simulink model "Model_IPS6"  (R2016a)
settings: Solver=VariableStepAuto  StartTime=0  StopTime=15
values from neighbouring files (symbols this model uses):
  Imrn = 7.4    [parametriAM.m]
  In = 12.7    [parametriAM.m]
  Ismax = In*sqrt(2)    [parametriAM.m]
  J = 0.019    [parametriAM.m]
  Ki_Imr = 1000    [parametriAM.m]
  Ki_tok = 5.0    (= 5)    [parametriAM.m]
  Ki_wr = 1000    [parametriAM.m]
  Kp_Imr = 100    [parametriAM.m]
  Kp_tok = 0.05    [parametriAM.m]
  Kp_wr = 50    [parametriAM.m]
  Lm = 0.0493    [parametriAM.m]
  Lr = 0.05315    [parametriAM.m]
  Ls = 0.05315    [parametriAM.m]
  Lst = sigma*Ls    (= 0.00742111947319)    [parametriAM.m]
  pp = 3    [parametriAM.m]
  Rs = 0.594    [parametriAM.m]
  sigma = 1 - 1/((1+sigmaR)*(1+sigmaS))    (= 0.13962595434)    [parametriAM.m]
  taufiltra = 1/(2*pi*fcutoff)    (= 1.59154943092e-05)    [parametriAM.m]
  Tr = Lr/Rr    (= 0.0771407837446)    [parametriAM.m]
  Udc = Un*sqrt(2)    [parametriAM.m]
  wb_upper_limit_field_weaking = sqrt((Ls^2+Lst^2)/(2*Lst^2*Ls^2))*Usmax/Ismax    [parametriAM.m]
  wdod = 2000*2*pi/60    (= 209.439510239)    [parametriAM.m]
libraries: simulink x20
(part 1 of 2)
settings Model: Creator=Vaje  LastModifiedBy=Mitja1

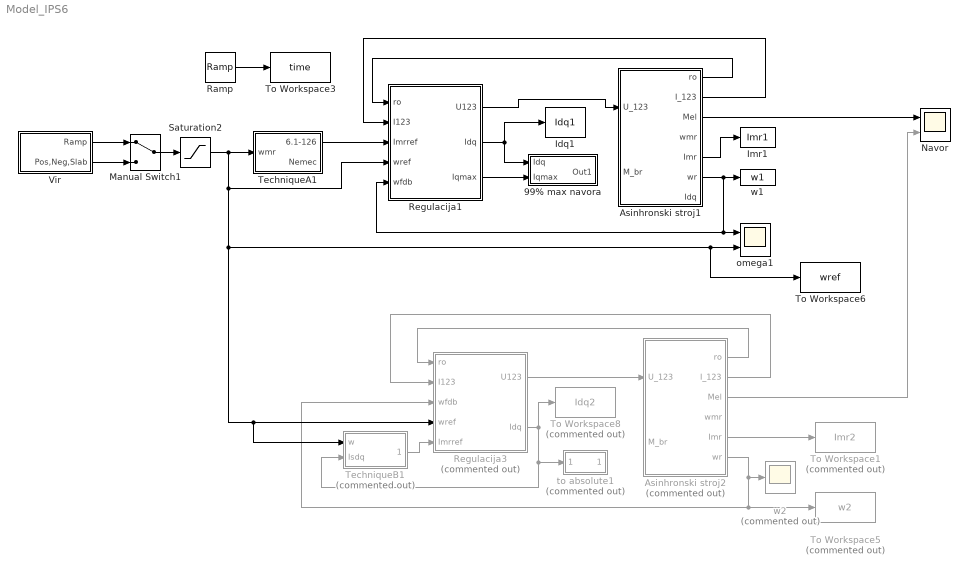
== system Model_IPS6 ==
  99% max navora : Subsystem
  Asinhronski stroj1 : Subsystem  InitFcn=parametriAM
  Asinhronski stroj2 : Subsystem  Commented=on  InitFcn=parametriAM
  Idq1 : ToWorkspace  VariableName=Idq1  SampleTime=-1
      settings: Decimation=3  Save2DSignal=2-D array (concatenate along first dimension)
  Imr1 : ToWorkspace  VariableName=Imr1  SampleTime=-1
      settings: Decimation=3  Save2DSignal=2-D array (concatenate along first dimension)
  Manual Switch1 : ManualSwitch
  Navor : Scope  NumInputPorts=2
  Ramp : simulink/Sources/Ramp  slope=1  start=0  X0=0
  Regulacija1 : Subsystem
  Regulacija3 : Subsystem  Commented=on
  Saturation2 : Saturate  UpperLimit=wb_upper_limit_field_weaking  LowerLimit=-wb_upper_limit_field_weaking
  TechniqueA1 : Subsystem
  TechniqueB1 : Subsystem  Commented=on
  To Workspace1 : ToWorkspace  Commented=on  VariableName=Imr2  SampleTime=-1
      settings: Decimation=3  Save2DSignal=2-D array (concatenate along first dimension)
  To Workspace3 : ToWorkspace  VariableName=time  SampleTime=-1
      settings: Decimation=3  Save2DSignal=2-D array (concatenate along first dimension)
  To Workspace5 : ToWorkspace  Commented=on  VariableName=w2  SampleTime=-1
      settings: Decimation=3  Save2DSignal=2-D array (concatenate along first dimension)
  To Workspace6 : ToWorkspace  VariableName=wref  SampleTime=-1
      settings: Decimation=3  Save2DSignal=2-D array (concatenate along first dimension)
  To Workspace8 : ToWorkspace  Commented=on  VariableName=Idq2  SampleTime=-1
      settings: Decimation=3  Save2DSignal=2-D array (concatenate along first dimension)
  Vir : Subsystem
  omega1 : Scope  NumInputPorts=2
  to absolute1 : Subsystem  Commented=on
  w1 : ToWorkspace  VariableName=w1  SampleTime=-1
      settings: Decimation=3  Save2DSignal=2-D array (concatenate along first dimension)
  w2 : Scope  Commented=on
  wires:
  Vir/1(Ramp) -> Manual Switch1/1
  Vir/2(Pos,Neg,Slab) -> Manual Switch1/2
  Asinhronski stroj1/5(Imr) -> Imr1/1
  Ramp/1 -> To Workspace3/1
  TechniqueA1/1(6.1-126) -> Regulacija1/3(Imrref)
  Regulacija1/2(Idq) -> Idq1/1, 99% max navora/1("\tIdq")
  Asinhronski stroj1/1(ro) -> Regulacija1/1(ro)
  Asinhronski stroj1/2(I_123) -> Regulacija1/2(I123)
  Regulacija1/1(U123) -> Asinhronski stroj1/1(U_123)
  Asinhronski stroj1/6(wr) -> omega1/1, Regulacija1/5(wfdb), w1/1
  Asinhronski stroj2/5(Imr) -> To Workspace1/1
  Manual Switch1/1 -> Saturation2/1
  Regulacija3/2(Idq) -> TechniqueB1/2(Isdq), to absolute1/1(In1), To Workspace8/1
  Asinhronski stroj2/1(ro) -> Regulacija3/1(ro)
  Asinhronski stroj2/2(I_123) -> Regulacija3/2(I123)
  Regulacija3/1(U123) -> Asinhronski stroj2/1(U_123)
  Asinhronski stroj2/6(wr) -> Regulacija3/3(wfdb), To Workspace5/1, w2/1
  TechniqueB1/1(6.1-135) -> Regulacija3/5(Imrref)
  Saturation2/1 -> TechniqueB1/1(w), Regulacija3/4(wref), To Workspace6/1, omega1/2, Regulacija1/4(wref), TechniqueA1/1(wmr)
  Regulacija1/3(Iqmax) -> 99% max navora/2(Iqmax)
  Asinhronski stroj1/3(Mel) -> Navor/1
  Asinhronski stroj2/3(Mel) -> Navor/2

== system Model_IPS6/99% max navora ==
  "\tIdq" : Inport
  Iqmax : Inport  Port=2
  Demux : Demux  Outputs=2
  Gain1 : Gain  Gain=3*pp/2
  Gain2 : Gain  Gain=Lm*Lm/Lr
  Product2 : Product  Inputs=3  RndMeth=Zero
  Step : Step  Time=0.6  After=0.99  SampleTime=0
  Out1 : Outport
  wires:
  "\tIdq"/1 -> Demux/1
  Demux/1 -> Product2/1
  Iqmax/1 -> Product2/2
  Step/1 -> Product2/3
  Gain1/1 -> Gain2/1
  Product2/1 -> Gain1/1
  Gain2/1 -> Out1/1

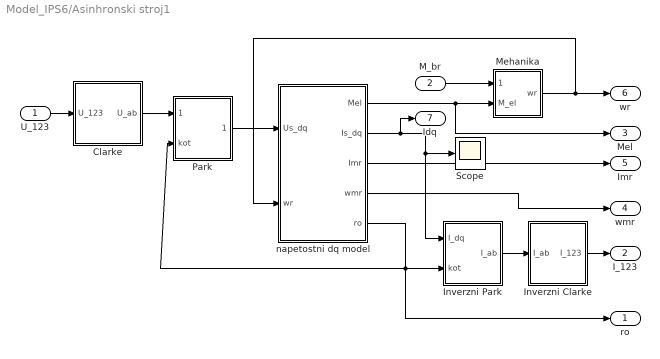
== system Model_IPS6/Asinhronski stroj1 ==
  U_123 : Inport
  M_br : Inport  Port=2
  Clarke : Subsystem
  Inverzni Clarke : Subsystem
  Inverzni Park : Subsystem
  Mehanika : Subsystem
  Park : Subsystem
  Scope : Scope
  napetostni dq model : Subsystem
  ro : Outport
  I_123 : Outport  Port=2
  Mel : Outport  Port=3
  wmr : Outport  Port=4
  Imr : Outport  Port=5
  wr : Outport  Port=6
  Idq : Outport  Port=7
  wires:
  Inverzni Park/1(I_ab) -> Inverzni Clarke/1(I_ab)
  Clarke/1(U_ab) -> Park/1(U_ab)
  Mehanika/1(wr) -> napetostni dq model/2(wr), wr/1
  M_br/1 -> Mehanika/1(M_br)
  napetostni dq model/1(Mel) -> Mel/1, Mehanika/2(M_el)
  Inverzni Clarke/1(I_123) -> I_123/1
  napetostni dq model/4(wmr) -> wmr/1
  napetostni dq model/3(Imr) -> Imr/1
  U_123/1 -> Clarke/1(U_123)
  napetostni dq model/2(Is_dq) -> Idq/1, Scope/1, Inverzni Park/1(I_dq)
  napetostni dq model/5(ro) -> ro/1, Park/2(kot), Inverzni Park/2(kot)
  Park/1(U_dq) -> napetostni dq model/1(Us_dq)

== system Model_IPS6/Asinhronski stroj2 ==
  U_123 : Inport
  M_br : Inport  Port=2
  Clarke : Subsystem
  Inverzni Clarke : Subsystem
  Inverzni Park : Subsystem
  Mehanika : Subsystem
  Park : Subsystem
  Scope : Scope
  napetostni dq model : Subsystem
  ro : Outport
  I_123 : Outport  Port=2
  Mel : Outport  Port=3
  wmr : Outport  Port=4
  Imr : Outport  Port=5
  wr : Outport  Port=6
  wires:
  Park/1(U_dq) -> napetostni dq model/1(Us_dq), Scope/1
  napetostni dq model/5(ro) -> Inverzni Park/2(kot), Park/2(kot), ro/1
  napetostni dq model/2(Is_dq) -> Inverzni Park/1(I_dq)
  U_123/1 -> Clarke/1(U_123)
  napetostni dq model/3(Imr) -> Imr/1
  napetostni dq model/4(wmr) -> wmr/1
  Inverzni Clarke/1(I_123) -> I_123/1
  napetostni dq model/1(Mel) -> Mehanika/2(M_el), Mel/1
  M_br/1 -> Mehanika/1(M_br)
  Mehanika/1(wr) -> wr/1, napetostni dq model/2(wr)
  Clarke/1(U_ab) -> Park/1(U_ab)
  Inverzni Park/1(I_ab) -> Inverzni Clarke/1(I_ab)

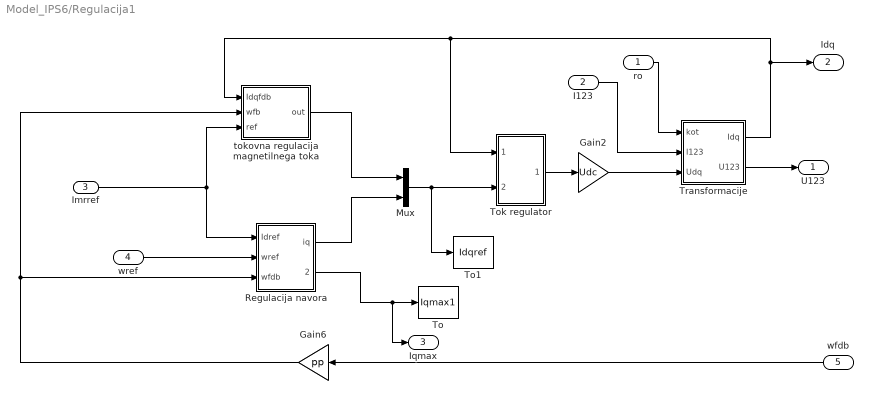
== system Model_IPS6/Regulacija1 ==
  ro : Inport
  I123 : Inport  Port=2
  Imrref : Inport  Port=3
  wref : Inport  Port=4
  wfdb : Inport  Port=5
  Gain2 : Gain  Gain=Udc
  Gain6 : Gain  Gain=pp
  Mux : Mux  Inputs=2
  Regulacija navora : Subsystem
  To : ToWorkspace  VariableName=Iqmax1  SampleTime=-1
      settings: Decimation=3  Save2DSignal=2-D array (concatenate along first dimension)
  To1 : ToWorkspace  VariableName=Idqref  SampleTime=-1
      settings: Decimation=3  Save2DSignal=2-D array (concatenate along first dimension)
  Tok regulator : Subsystem
  Transformacije : Subsystem
  tokovna regulacija magnetilnega toka : Subsystem
  U123 : Outport
  Idq : Outport  Port=2
  Iqmax : Outport  Port=3
  wires:
  Imrref/1 -> Regulacija navora/1(Idref), tokovna regulacija magnetilnega toka/3(ref)
  wref/1 -> Regulacija navora/2(wref)
  Transformacije/1(Idq) -> Tok regulator/1(Idqdej), tokovna regulacija magnetilnega toka/1(Idqfdb), Idq/1
  ro/1 -> Transformacije/1(kot)
  I123/1 -> Transformacije/2(I123)
  Gain2/1 -> Transformacije/3(Udq)
  wfdb/1 -> Gain6/1
  tokovna regulacija magnetilnega toka/1(out) -> Mux/1
  Mux/1 -> To1/1, Tok regulator/2(Idqref)
  Tok regulator/1(Udq) -> Gain2/1
  Regulacija navora/1(iq) -> Mux/2
  Transformacije/2(U123) -> U123/1
  Regulacija navora/2(Iqmax) -> Iqmax/1, To/1
  Gain6/1 -> tokovna regulacija magnetilnega toka/2(wfb), Regulacija navora/3(wfdb)

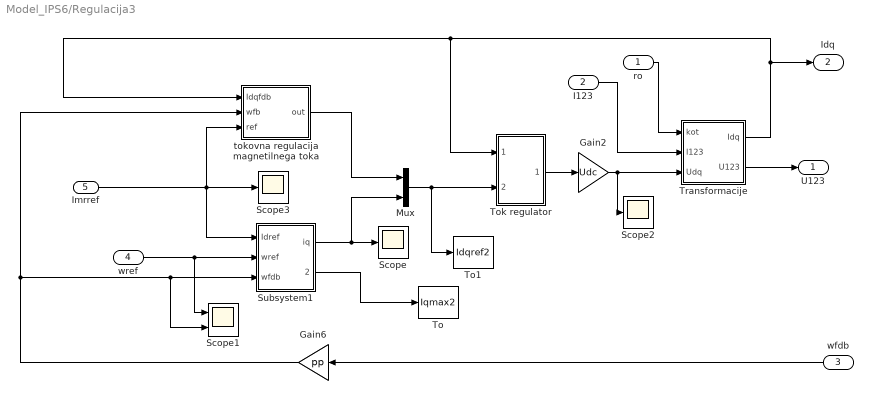
== system Model_IPS6/Regulacija3 ==
  ro : Inport
  I123 : Inport  Port=2
  wfdb : Inport  Port=3
  wref : Inport  Port=4
  Imrref : Inport  Port=5
  Gain2 : Gain  Gain=Udc
  Gain6 : Gain  Gain=pp
  Mux : Mux  Inputs=2
  Scope : Scope
  Scope1 : Scope  NumInputPorts=2
  Scope2 : Scope
  Scope3 : Scope
  Subsystem1 : Subsystem
  To : ToWorkspace  VariableName=Iqmax2  SampleTime=-1
      settings: Decimation=3  Save2DSignal=2-D array (concatenate along first dimension)
  To1 : ToWorkspace  VariableName=Idqref2  SampleTime=-1
      settings: Decimation=3  Save2DSignal=2-D array (concatenate along first dimension)
  Tok regulator : Subsystem
  Transformacije : Subsystem
  tokovna regulacija magnetilnega toka : Subsystem
  U123 : Outport
  Idq : Outport  Port=2
  wires:
  Gain6/1 -> Subsystem1/3(wfdb), Scope1/2, tokovna regulacija magnetilnega toka/2(wfb)
  Subsystem1/2(Iqmax) -> To/1
  Transformacije/2(U123) -> U123/1
  Subsystem1/1(iq) -> Mux/2, Scope/1
  Tok regulator/1(Udq) -> Gain2/1
  Mux/1 -> Tok regulator/2(Idqref), To1/1
  tokovna regulacija magnetilnega toka/1(out) -> Mux/1
  wfdb/1 -> Gain6/1
  Gain2/1 -> Transformacije/3(Udq), Scope2/1
  I123/1 -> Transformacije/2(I123)
  ro/1 -> Transformacije/1(kot)
  Transformacije/1(Idq) -> Idq/1, tokovna regulacija magnetilnega toka/1(Idqfdb), Tok regulator/1(Idqdej)
  wref/1 -> Scope1/1, Subsystem1/2(wref)
  Imrref/1 -> tokovna regulacija magnetilnega toka/3(ref), Scope3/1, Subsystem1/1(Idref)

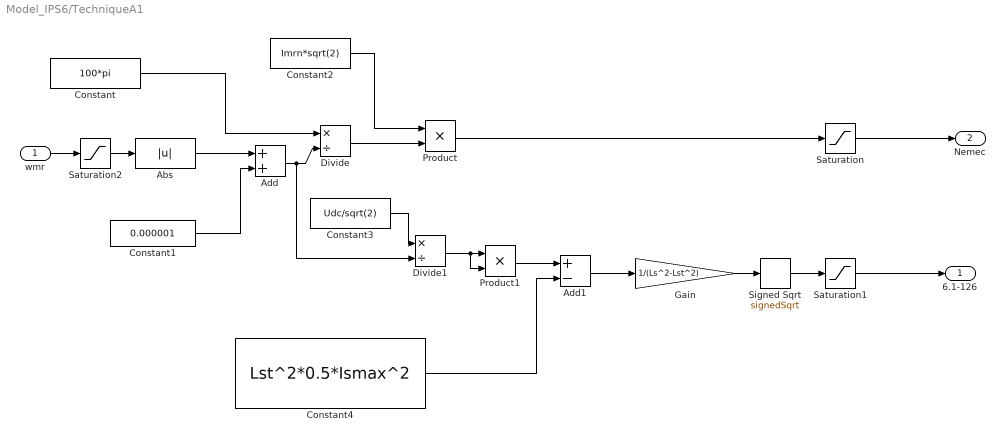
== system Model_IPS6/TechniqueA1 ==
  wmr : Inport
  Abs : Abs
  Add : Sum
  Add1 : Sum  Inputs=+-
  Constant : Constant  Value=100*pi
  Constant1 : Constant  Value=0.000001
  Constant2 : Constant  Value=Imrn*sqrt(2)
  Constant3 : Constant  Value=Udc/sqrt(2)
  Constant4 : Constant  Value=Lst^2*0.5*Ismax^2
  Divide : Product  Inputs=*/
  Divide1 : Product  Inputs=*/
  Gain : Gain  Gain=1/(Ls^2-Lst^2)
  Product : Product
  Product1 : Product
  Saturation : Saturate  UpperLimit=+Imrn*sqrt(2)  LowerLimit=0
  Saturation1 : Saturate  UpperLimit=+Imrn*sqrt(2)  LowerLimit=-Imrn*sqrt(2)
  Saturation2 : Saturate  UpperLimit=wb_upper_limit_field_weaking  LowerLimit=-wb_upper_limit_field_weaking
  Signed Sqrt : Sqrt  Operator=signedSqrt  SaturateOnIntegerOverflow=on
  6.1-126 : Outport
  Nemec : Outport  Port=2
  wires:
  Constant2/1 -> Product/1
  Divide/1 -> Product/2
  Product/1 -> Saturation/1
  Constant/1 -> Divide/1
  Add/1 -> Divide1/2, Divide/2
  Abs/1 -> Add/1
  Constant1/1 -> Add/2
  Saturation/1 -> Nemec/1
  Constant3/1 -> Divide1/1
  Divide1/1 -> Product1/2, Product1/1
  Product1/1 -> Add1/1
  Constant4/1 -> Add1/2
  Saturation1/1 -> 6.1-126/1
  Add1/1 -> Gain/1
  Gain/1 -> Signed Sqrt/1
  Signed Sqrt/1 -> Saturation1/1
  wmr/1 -> Saturation2/1
  Saturation2/1 -> Abs/1

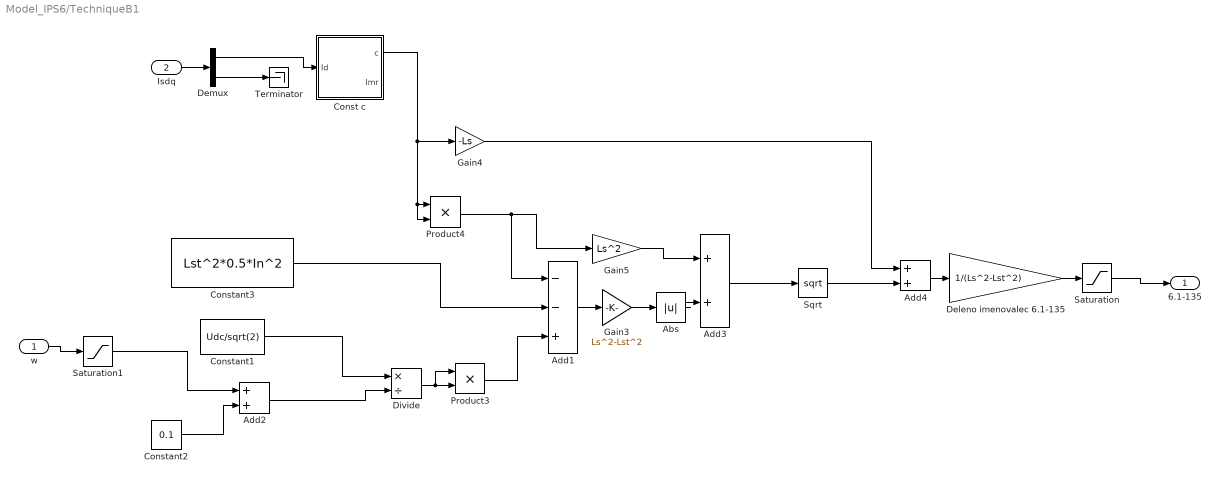
== system Model_IPS6/TechniqueB1 ==
  w : Inport
  Isdq : Inport  Port=2
  Abs : Abs
  Add1 : Sum  Inputs=--+
  Add2 : Sum
  Add3 : Sum
  Add4 : Sum
  Const c : Subsystem
  Constant1 : Constant  Value=Udc/sqrt(2)
  Constant2 : Constant  Value=0.1
  Constant3 : Constant  Value=Lst^2*0.5*In^2
  Deleno imenovalec 6.1-135 : Gain  Gain=1/(Ls^2-Lst^2)
  Demux : Demux  Outputs=2
  Divide : Product  Inputs=*/
  Gain3 : Gain  Gain=Ls^2-Lst^2
  Gain4 : Gain  Gain=-Ls
  Gain5 : Gain  Gain=Ls^2
  Product3 : Product
  Product4 : Product
  Saturation : Saturate  UpperLimit=+Imrn*sqrt(2)  LowerLimit=-Imrn*sqrt(2)
  Saturation1 : Saturate  UpperLimit=wb_upper_limit_field_weaking  LowerLimit=-wb_upper_limit_field_weaking
  Sqrt : Sqrt  SaturateOnIntegerOverflow=on
  Terminator : Terminator
  6.1-135 : Outport
  wires:
  Constant1/1 -> Divide/1
  w/1 -> Saturation1/1
  Constant2/1 -> Add2/2
  Demux/1 -> Const c/1(Id)
  Demux/2 -> Terminator/1
  Saturation/1 -> 6.1-135/1
  Const c/1(c) -> Product4/2, Product4/1, Gain4/1
  Product4/1 -> Add1/1, Gain5/1
  Gain5/1 -> Add3/1
  Gain4/1 -> Add4/1
  Add4/1 -> Deleno imenovalec 6.1-135/1
  Deleno imenovalec 6.1-135/1 -> Saturation/1
  Add1/1 -> Gain3/1
  Constant3/1 -> Add1/2
  Add2/1 -> Divide/2
  Divide/1 -> Product3/1, Product3/2
  Product3/1 -> Add1/3
  Sqrt/1 -> Add4/2
  Gain3/1 -> Abs/1
  Add3/1 -> Sqrt/1
  Abs/1 -> Add3/2
  Saturation1/1 -> Add2/1
  Isdq/1 -> Demux/1

== system Model_IPS6/Vir ==
  Add1 : Sum  Inputs=++++++
  Rampa : simulink/Sources/Ramp  slope=500*2*pi/60  start=0.5  X0=0
  Step : Step  Time=0.2  After=2000*2*pi/60  SampleTime=0
  Step1 : Step  Time=0.4  After=1000*pi/30  SampleTime=0
  Step2 : Step  Time=2  After=2000*2*pi/60  SampleTime=0
  Step3 : Step  Time=3  After=2000*2*pi/60  SampleTime=0
  Step4 : Step  Time=8  After=wdod  SampleTime=0
  Step5 : Step  Time=9  After=wdod  SampleTime=0
  Ramp : Outport
  Pos,Neg,Slab : Outport  Port=2
  wires:
  Add1/1 -> Pos,Neg,Slab/1
  Step/1 -> Add1/1
  Rampa/1 -> Ramp/1
  Step1/1 -> Add1/2

== system Model_IPS6/to absolute1 ==
  In1 : Inport
  Abs1 : Abs
  Demux : Demux  Outputs=2
  Real-Imag to Complex1 : RealImagToComplex
  Out1 : Outport
  wires:
  Demux/2 -> Real-Imag to Complex1/2
  Demux/1 -> Real-Imag to Complex1/1
  In1/1 -> Demux/1
  Abs1/1 -> Out1/1
  Real-Imag to Complex1/1 -> Abs1/1

== system Model_IPS6/Asinhronski stroj1/Clarke ==
  U_123 : Inport
  ABC_ab1 : Subsystem
  Demux : Demux  Outputs=3
  Mux : Mux  Inputs=2
  U_ab : Outport
  wires:
  Mux/1 -> U_ab/1
  ABC_ab1/2(beta) -> Mux/2
  ABC_ab1/1(alfa) -> Mux/1
  Demux/3 -> ABC_ab1/3(C)
  Demux/2 -> ABC_ab1/2(B)
  Demux/1 -> ABC_ab1/1(A)
  U_123/1 -> Demux/1

== system Model_IPS6/Asinhronski stroj1/Inverzni Clarke ==
  I_ab : Inport
  Demux : Demux  Outputs=2
  Mux : Mux  Inputs=3
  ab_ABC : Subsystem
  I_123 : Outport
  wires:
  ab_ABC/3(C) -> Mux/3
  ab_ABC/2(B) -> Mux/2
  ab_ABC/1(A) -> Mux/1
  Demux/2 -> ab_ABC/2(beta)
  Demux/1 -> ab_ABC/1(alfa)
  I_ab/1 -> Demux/1
  Mux/1 -> I_123/1

== system Model_IPS6/Asinhronski stroj1/Inverzni Park ==
  I_dq : Inport
  kot : Inport  Port=2
  Demux : Demux  Outputs=2
  Mux : Mux  Inputs=2
  "Sum1 " : Sum  Inputs=+-  SaturateOnIntegerOverflow=on  InputSameDT=on  OutDataTypeStr=Inherit: Same as first input
  Sum2 : Sum  SaturateOnIntegerOverflow=on  InputSameDT=on  OutDataTypeStr=Inherit: Same as first input
  cos : Fcn  Expr=cos(u)
  sin : Fcn  Expr=sin(u)
  x_d*cos : Product  SaturateOnIntegerOverflow=on  RndMeth=Zero  InputSameDT=on  OutDataTypeStr=Inherit: Same as first input
  x_d*sin : Product  SaturateOnIntegerOverflow=on  RndMeth=Zero  InputSameDT=on  OutDataTypeStr=Inherit: Same as first input
  x_q*cos : Product  SaturateOnIntegerOverflow=on  RndMeth=Zero  InputSameDT=on  OutDataTypeStr=Inherit: Same as first input
  "x_q*sin " : Product  SaturateOnIntegerOverflow=on  RndMeth=Zero  InputSameDT=on  OutDataTypeStr=Inherit: Same as first input
  I_ab : Outport
  wires:
  Mux/1 -> I_ab/1
  I_dq/1 -> Demux/1
  Demux/1 -> x_d*sin/1, x_d*cos/1
  Demux/2 -> "x_q*sin "/1, x_q*cos/1
  cos/1 -> x_q*cos/2, x_d*cos/2
  sin/1 -> "x_q*sin "/2, x_d*sin/2
  x_d*cos/1 -> "Sum1 "/1
  "x_q*sin "/1 -> "Sum1 "/2
  x_q*cos/1 -> Sum2/2
  x_d*sin/1 -> Sum2/1
  "Sum1 "/1 -> Mux/1
  Sum2/1 -> Mux/2
  kot/1 -> cos/1, sin/1

== system Model_IPS6/Asinhronski stroj1/Mehanika ==
  M_br : Inport
  M_el : Inport  Port=2
  Sum : Sum  Inputs=+-
  eq 2.19 : Subsystem
  wr : Outport
  wires:
  M_br/1 -> Sum/2
  Sum/1 -> eq 2.19/1(M)
  M_el/1 -> Sum/1
  eq 2.19/1(wr) -> wr/1

== system Model_IPS6/Asinhronski stroj1/Park ==
  U_ab : Inport
  kot : Inport  Port=2
  Demux : Demux  Outputs=2
  Mux : Mux  Inputs=2
  "Sum1 " : Sum  SaturateOnIntegerOverflow=on  InputSameDT=on  OutDataTypeStr=Inherit: Same as first input
  Sum2 : Sum  Inputs=-+  SaturateOnIntegerOverflow=on  InputSameDT=on  OutDataTypeStr=Inherit: Same as first input
  cos : Fcn  Expr=cos(u)
  sin : Fcn  Expr=sin(u)
  x_a*cos : Product  SaturateOnIntegerOverflow=on  RndMeth=Zero  InputSameDT=on  OutDataTypeStr=Inherit: Same as first input
  x_a*sin : Product  SaturateOnIntegerOverflow=on  RndMeth=Zero  InputSameDT=on  OutDataTypeStr=Inherit: Same as first input
  x_b*cos : Product  SaturateOnIntegerOverflow=on  RndMeth=Zero  InputSameDT=on  OutDataTypeStr=Inherit: Same as first input
  "x_b*sin " : Product  SaturateOnIntegerOverflow=on  RndMeth=Zero  InputSameDT=on  OutDataTypeStr=Inherit: Same as first input
  U_dq : Outport
  wires:
  Mux/1 -> U_dq/1
  U_ab/1 -> Demux/1
  Demux/1 -> x_a*sin/1, x_a*cos/1
  Demux/2 -> "x_b*sin "/1, x_b*cos/1
  cos/1 -> x_b*cos/2, x_a*cos/2
  sin/1 -> "x_b*sin "/2, x_a*sin/2
  x_a*cos/1 -> "Sum1 "/1
  "x_b*sin "/1 -> "Sum1 "/2
  x_b*cos/1 -> Sum2/2
  x_a*sin/1 -> Sum2/1
  "Sum1 "/1 -> Mux/1
  Sum2/1 -> Mux/2
  kot/1 -> cos/1, sin/1

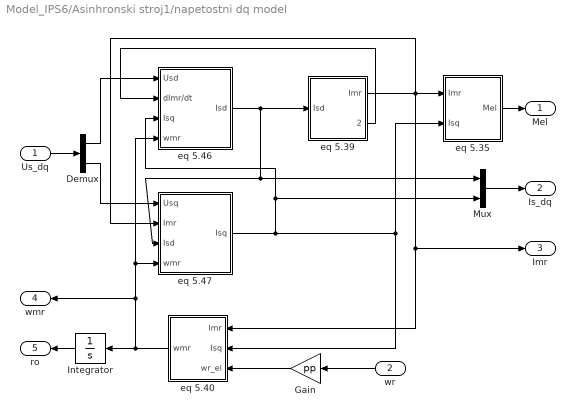
== system Model_IPS6/Asinhronski stroj1/napetostni dq model ==
  Us_dq : Inport
  wr : Inport  Port=2
  Demux : Demux  Outputs=2
  Gain : Gain  Gain=pp
  Integrator : Integrator
  Mux : Mux  Inputs=2
  eq 5.35 : Subsystem
  eq 5.39 : Subsystem
  eq 5.40 : Subsystem
  eq 5.46 : Subsystem
  eq 5.47 : Subsystem
  Mel : Outport
  Is_dq : Outport  Port=2
  Imr : Outport  Port=3
  wmr : Outport  Port=4
  ro : Outport  Port=5
  wires:
  Gain/1 -> eq 5.40/3(wr_el)
  Mux/1 -> Is_dq/1
  Demux/2 -> eq 5.47/1(Usq)
  Demux/1 -> eq 5.46/1(Usd)
  Us_dq/1 -> Demux/1
  wr/1 -> Gain/1
  Integrator/1 -> ro/1
  eq 5.35/1(Mel) -> Mel/1
  eq 5.40/1(wmr) -> Integrator/1, wmr/1, eq 5.46/4(wmr), eq 5.47/4(wmr)
  eq 5.47/1(Isq) -> Mux/2, eq 5.46/3(Isq), eq 5.40/2(Isq), eq 5.35/2(Isq)
  eq 5.39/1(Imr) -> eq 5.47/2(Imr), Imr/1, eq 5.40/1(Imr), eq 5.35/1(Imr)
  eq 5.39/2(dImr/dt) -> eq 5.46/2(dImr/dt)
  eq 5.46/1(Isd) -> Mux/1, eq 5.47/3(Isd), eq 5.39/1(Isd)

== system Model_IPS6/Asinhronski stroj2/Clarke ==
  U_123 : Inport
  ABC_ab1 : Subsystem
  Demux : Demux  Outputs=3
  Mux : Mux  Inputs=2
  U_ab : Outport
  wires:
  U_123/1 -> Demux/1
  Demux/1 -> ABC_ab1/1(A)
  Demux/2 -> ABC_ab1/2(B)
  Demux/3 -> ABC_ab1/3(C)
  ABC_ab1/1(alfa) -> Mux/1
  ABC_ab1/2(beta) -> Mux/2
  Mux/1 -> U_ab/1

== system Model_IPS6/Asinhronski stroj2/Inverzni Clarke ==
  I_ab : Inport
  Demux : Demux  Outputs=2
  Mux : Mux  Inputs=3
  ab_ABC : Subsystem
  I_123 : Outport
  wires:
  Mux/1 -> I_123/1
  I_ab/1 -> Demux/1
  Demux/1 -> ab_ABC/1(alfa)
  Demux/2 -> ab_ABC/2(beta)
  ab_ABC/1(A) -> Mux/1
  ab_ABC/2(B) -> Mux/2
  ab_ABC/3(C) -> Mux/3

== system Model_IPS6/Asinhronski stroj2/Inverzni Park ==
  I_dq : Inport
  kot : Inport  Port=2
  Demux : Demux  Outputs=2
  Mux : Mux  Inputs=2
  "Sum1 " : Sum  Inputs=+-  SaturateOnIntegerOverflow=on  InputSameDT=on  OutDataTypeStr=Inherit: Same as first input
  Sum2 : Sum  SaturateOnIntegerOverflow=on  InputSameDT=on  OutDataTypeStr=Inherit: Same as first input
  cos : Fcn  Expr=cos(u)
  sin : Fcn  Expr=sin(u)
  x_d*cos : Product  SaturateOnIntegerOverflow=on  RndMeth=Zero  InputSameDT=on  OutDataTypeStr=Inherit: Same as first input
  x_d*sin : Product  SaturateOnIntegerOverflow=on  RndMeth=Zero  InputSameDT=on  OutDataTypeStr=Inherit: Same as first input
  x_q*cos : Product  SaturateOnIntegerOverflow=on  RndMeth=Zero  InputSameDT=on  OutDataTypeStr=Inherit: Same as first input
  "x_q*sin " : Product  SaturateOnIntegerOverflow=on  RndMeth=Zero  InputSameDT=on  OutDataTypeStr=Inherit: Same as first input
  I_ab : Outport
  wires:
  kot/1 -> sin/1, cos/1
  Sum2/1 -> Mux/2
  "Sum1 "/1 -> Mux/1
  x_d*sin/1 -> Sum2/1
  x_q*cos/1 -> Sum2/2
  "x_q*sin "/1 -> "Sum1 "/2
  x_d*cos/1 -> "Sum1 "/1
  sin/1 -> x_d*sin/2, "x_q*sin "/2
  cos/1 -> x_d*cos/2, x_q*cos/2
  Demux/2 -> x_q*cos/1, "x_q*sin "/1
  Demux/1 -> x_d*cos/1, x_d*sin/1
  I_dq/1 -> Demux/1
  Mux/1 -> I_ab/1

== system Model_IPS6/Asinhronski stroj2/Mehanika ==
  M_br : Inport
  M_el : Inport  Port=2
  Sum : Sum  Inputs=+-
  eq 2.19 : Subsystem
  wr : Outport
  wires:
  eq 2.19/1(wr) -> wr/1
  M_el/1 -> Sum/1
  Sum/1 -> eq 2.19/1(M)
  M_br/1 -> Sum/2

== system Model_IPS6/Asinhronski stroj2/Park ==
  U_ab : Inport
  kot : Inport  Port=2
  Demux : Demux  Outputs=2
  Mux : Mux  Inputs=2
  "Sum1 " : Sum  SaturateOnIntegerOverflow=on  InputSameDT=on  OutDataTypeStr=Inherit: Same as first input
  Sum2 : Sum  Inputs=-+  SaturateOnIntegerOverflow=on  InputSameDT=on  OutDataTypeStr=Inherit: Same as first input
  cos : Fcn  Expr=cos(u)
  sin : Fcn  Expr=sin(u)
  x_a*cos : Product  SaturateOnIntegerOverflow=on  RndMeth=Zero  InputSameDT=on  OutDataTypeStr=Inherit: Same as first input
  x_a*sin : Product  SaturateOnIntegerOverflow=on  RndMeth=Zero  InputSameDT=on  OutDataTypeStr=Inherit: Same as first input
  x_b*cos : Product  SaturateOnIntegerOverflow=on  RndMeth=Zero  InputSameDT=on  OutDataTypeStr=Inherit: Same as first input
  "x_b*sin " : Product  SaturateOnIntegerOverflow=on  RndMeth=Zero  InputSameDT=on  OutDataTypeStr=Inherit: Same as first input
  U_dq : Outport
  wires:
  kot/1 -> sin/1, cos/1
  Sum2/1 -> Mux/2
  "Sum1 "/1 -> Mux/1
  x_a*sin/1 -> Sum2/1
  x_b*cos/1 -> Sum2/2
  "x_b*sin "/1 -> "Sum1 "/2
  x_a*cos/1 -> "Sum1 "/1
  sin/1 -> x_a*sin/2, "x_b*sin "/2
  cos/1 -> x_a*cos/2, x_b*cos/2
  Demux/2 -> x_b*cos/1, "x_b*sin "/1
  Demux/1 -> x_a*cos/1, x_a*sin/1
  U_ab/1 -> Demux/1
  Mux/1 -> U_dq/1

== system Model_IPS6/Asinhronski stroj2/napetostni dq model ==
  Us_dq : Inport
  wr : Inport  Port=2
  Demux : Demux  Outputs=2
  Gain : Gain  Gain=pp
  Integrator : Integrator
  Mux : Mux  Inputs=2
  eq 5.35 : Subsystem
  eq 5.39 : Subsystem
  eq 5.40 : Subsystem
  eq 5.46 : Subsystem
  eq 5.47 : Subsystem
  Mel : Outport
  Is_dq : Outport  Port=2
  Imr : Outport  Port=3
  wmr : Outport  Port=4
  ro : Outport  Port=5
  wires:
  eq 5.46/1(Isd) -> eq 5.39/1(Isd), eq 5.47/3(Isd), Mux/1
  eq 5.39/2(dImr/dt) -> eq 5.46/2(dImr/dt)
  eq 5.39/1(Imr) -> eq 5.35/1(Imr), eq 5.40/1(Imr), Imr/1, eq 5.47/2(Imr)
  eq 5.47/1(Isq) -> eq 5.35/2(Isq), eq 5.40/2(Isq), eq 5.46/3(Isq), Mux/2
  eq 5.40/1(wmr) -> eq 5.47/4(wmr), eq 5.46/4(wmr), wmr/1, Integrator/1
  eq 5.35/1(Mel) -> Mel/1
  Integrator/1 -> ro/1
  wr/1 -> Gain/1
  Us_dq/1 -> Demux/1
  Demux/1 -> eq 5.46/1(Usd)
  Demux/2 -> eq 5.47/1(Usq)
  Mux/1 -> Is_dq/1
  Gain/1 -> eq 5.40/3(wr_el)

== system Model_IPS6/Regulacija1/Regulacija navora ==
  Idref : Inport
  wref : Inport  Port=2
  wfdb : Inport  Port=3
  1/Ti : Gain  Gain=Ki_wr  SaturateOnIntegerOverflow=on  OutDataTypeStr=Inherit: Same as input  ParamDataTypeStr=Inherit: Same as input
  Abs : Abs
  Add2 : Sum  Inputs=+-
  Compare To Zero : simulink/Logic and Bit Operations/Compare To Zero  relop=<=  OutDataTypeStr=boolean
  Integrator : Integrator
  Kp : Gain  Gain=Kp_wr  SaturateOnIntegerOverflow=on  OutDataTypeStr=Inherit: Same as input  ParamDataTypeStr=Inherit: Same as input
  Limita q toka : Subsystem
  Product : Product
  Sum1 : Sum  Inputs=|+-
  Sum2 : Sum  Inputs=|++
  iq : Outport
  Iqmax : Outport  Port=2
  wires:
  1/Ti/1 -> Integrator/1
  Sum1/1 -> Product/1, Kp/1
  Integrator/1 -> Sum2/2
  Add2/1 -> Abs/1
  Abs/1 -> Compare To Zero/1
  Kp/1 -> Sum2/1
  Compare To Zero/1 -> Product/2
  Product/1 -> 1/Ti/1
  wref/1 -> Sum1/1
  wfdb/1 -> Limita q toka/2(w), Sum1/2
  Sum2/1 -> Limita q toka/3(Iq), Add2/1
  Limita q toka/2(Iq_lim) -> Add2/2, iq/1
  Idref/1 -> Limita q toka/1(Idref)
  Limita q toka/1(Out1) -> Iqmax/1

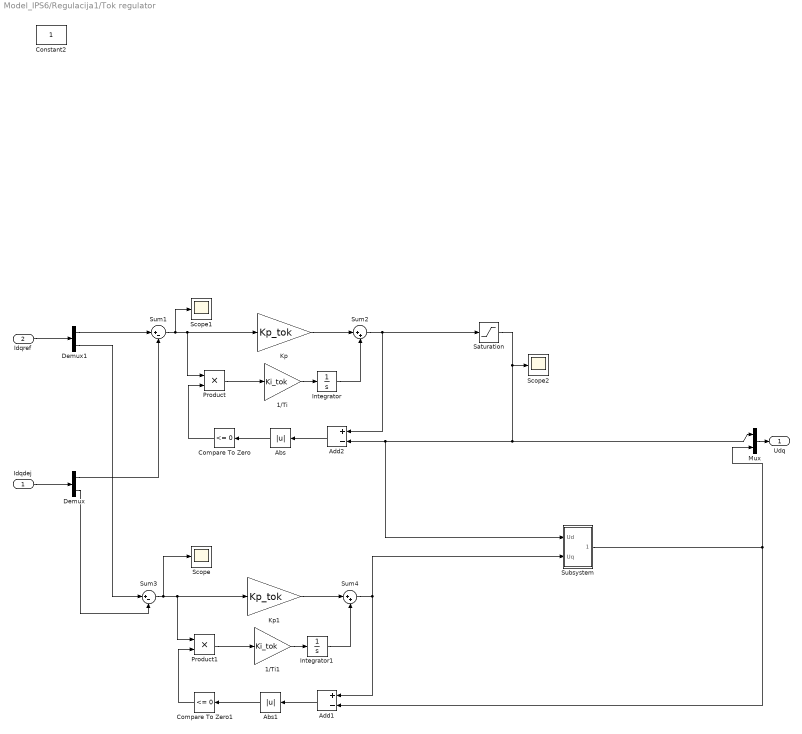
== system Model_IPS6/Regulacija1/Tok regulator ==
  Idqdej : Inport
  Idqref : Inport  Port=2
  1/Ti : Gain  Gain=Ki_tok  SaturateOnIntegerOverflow=on  OutDataTypeStr=Inherit: Same as input  ParamDataTypeStr=Inherit: Same as input
  1/Ti1 : Gain  Gain=Ki_tok  SaturateOnIntegerOverflow=on  OutDataTypeStr=Inherit: Same as input  ParamDataTypeStr=Inherit: Same as input
  Abs : Abs  ZeroCross=off
  Abs1 : Abs
  Add1 : Sum  Inputs=+-
  Add2 : Sum  Inputs=+-
  Compare To Zero : simulink/Logic and Bit Operations/Compare To Zero  relop=<=  OutDataTypeStr=boolean  ZeroCross=off
  Compare To Zero1 : simulink/Logic and Bit Operations/Compare To Zero  relop=<=  OutDataTypeStr=boolean
  Constant2 : Constant
  Demux : Demux  Outputs=2
  Demux1 : Demux  Outputs=2
  Integrator : Integrator
  Integrator1 : Integrator
  Kp : Gain  Gain=Kp_tok  SaturateOnIntegerOverflow=on  OutDataTypeStr=Inherit: Same as input  ParamDataTypeStr=Inherit: Same as input
  Kp1 : Gain  Gain=Kp_tok  SaturateOnIntegerOverflow=on  OutDataTypeStr=Inherit: Same as input  ParamDataTypeStr=Inherit: Same as input
  Mux : Mux  Inputs=2
  Product : Product
  Product1 : Product
  Saturation : Saturate  UpperLimit=0.990  LowerLimit=-0.990  ZeroCross=off
  Scope : Scope
  Scope1 : Scope
  Scope2 : Scope
  Subsystem : Subsystem
  Sum1 : Sum  Inputs=|+-
  Sum2 : Sum  Inputs=|++
  Sum3 : Sum  Inputs=|+-
  Sum4 : Sum  Inputs=|++
  Udq : Outport
  wires:
  Abs1/1 -> Compare To Zero1/1
  Add1/1 -> Abs1/1
  Compare To Zero1/1 -> Product1/2
  Product1/1 -> 1/Ti1/1
  Integrator1/1 -> Sum4/2
  Kp1/1 -> Sum4/1
  1/Ti1/1 -> Integrator1/1
  Sum3/1 -> Scope/1, Kp1/1, Product1/1
  Demux1/2 -> Sum3/1
  Idqref/1 -> Demux1/1
  Mux/1 -> Udq/1
  Sum1/1 -> Scope1/1, Product/1, Kp/1
  Integrator/1 -> Sum2/2
  Kp/1 -> Sum2/1
  Demux1/1 -> Sum1/1
  1/Ti/1 -> Integrator/1
  Add2/1 -> Abs/1
  Abs/1 -> Compare To Zero/1
  Compare To Zero/1 -> Product/2
  Product/1 -> 1/Ti/1
  Idqdej/1 -> Demux/1
  Demux/2 -> Sum3/2
  Demux/1 -> Sum1/2
  Saturation/1 -> Scope2/1, Mux/1, Subsystem/1(Ud), Add2/2
  Sum4/1 -> Add1/1, Subsystem/2(Uq)
  Sum2/1 -> Saturation/1, Add2/1
  Subsystem/1(Uq_lim) -> Add1/2, Mux/2

== system Model_IPS6/Regulacija1/Transformacije ==
  kot : Inport
  I123 : Inport  Port=2
  Udq : Inport  Port=3
  Clarke : Subsystem
  Inverzni Clarke : Subsystem
  Inverzni Park : Subsystem
  Park : Subsystem
  Idq : Outport
  U123 : Outport  Port=2
  wires:
  Inverzni Clarke/1(U_123) -> U123/1
  Park/1(I_dq) -> Idq/1
  kot/1 -> Park/2(kot), Inverzni Park/1(kot)
  Clarke/1(I_ab) -> Park/1(I_ab)
  Inverzni Park/1(U_ab) -> Inverzni Clarke/1(U_ab)
  Udq/1 -> Inverzni Park/2(U_dq)
  I123/1 -> Clarke/1(I_123)

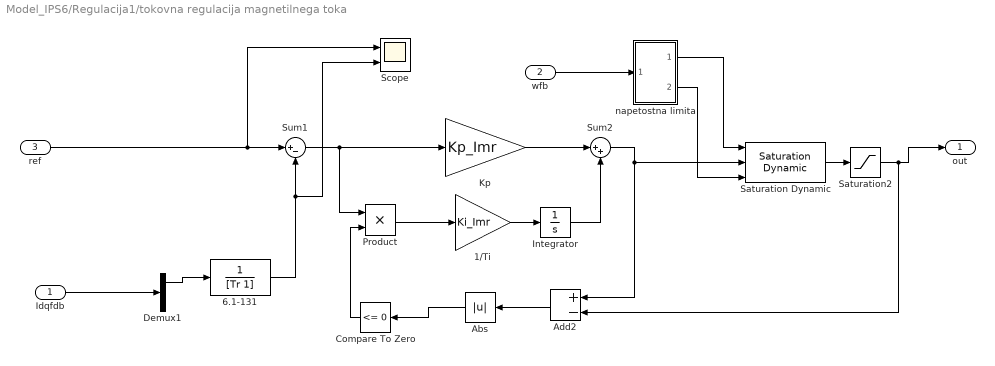
== system Model_IPS6/Regulacija1/tokovna regulacija magnetilnega toka ==
  Idqfdb : Inport
  wfb : Inport  Port=2
  ref : Inport  Port=3
  1/Ti : Gain  Gain=Ki_Imr  SaturateOnIntegerOverflow=on  OutDataTypeStr=Inherit: Same as input  ParamDataTypeStr=Inherit: Same as input
  6.1-131 : TransferFcn  Denominator=[Tr 1]
  Abs : Abs
  Add2 : Sum  Inputs=+-
  Compare To Zero : simulink/Logic and Bit Operations/Compare To Zero  relop=<=  OutDataTypeStr=boolean
  Demux1 : Demux  Outputs=2
  Integrator : Integrator
  Kp : Gain  Gain=Kp_Imr  SaturateOnIntegerOverflow=on  OutDataTypeStr=Inherit: Same as input  ParamDataTypeStr=Inherit: Same as input
  Product : Product
  Saturation Dynamic : simulink/Discontinuities/Saturation Dynamic  OutMin=[]  OutMax=[]  OutDataTypeStr=Inherit: Same as second input  OutDataType=fixdt(1, 16)  OutScaling=2^-10  DoSatur=off
  Saturation2 : Saturate  UpperLimit=Ismax  LowerLimit=-Ismax
  Scope : Scope  NumInputPorts=2
  Sum1 : Sum  Inputs=|+-
  Sum2 : Sum  Inputs=|++
  napetostna limita : Subsystem
  out : Outport
  wires:
  Product/1 -> 1/Ti/1
  Compare To Zero/1 -> Product/2
  Abs/1 -> Compare To Zero/1
  Add2/1 -> Abs/1
  Sum2/1 -> Add2/1, Saturation Dynamic/2
  Integrator/1 -> Sum2/2
  ref/1 -> Scope/1, Sum1/1
  Sum1/1 -> Kp/1, Product/1
  1/Ti/1 -> Integrator/1
  Kp/1 -> Sum2/1
  Demux1/1 -> 6.1-131/1
  6.1-131/1 -> Scope/2, Sum1/2
  Idqfdb/1 -> Demux1/1
  wfb/1 -> napetostna limita/1(wfb)
  napetostna limita/1(Out1) -> Saturation Dynamic/1
  napetostna limita/2(Out2) -> Saturation Dynamic/3
  Saturation Dynamic/1 -> Saturation2/1
  Saturation2/1 -> Add2/2, out/1

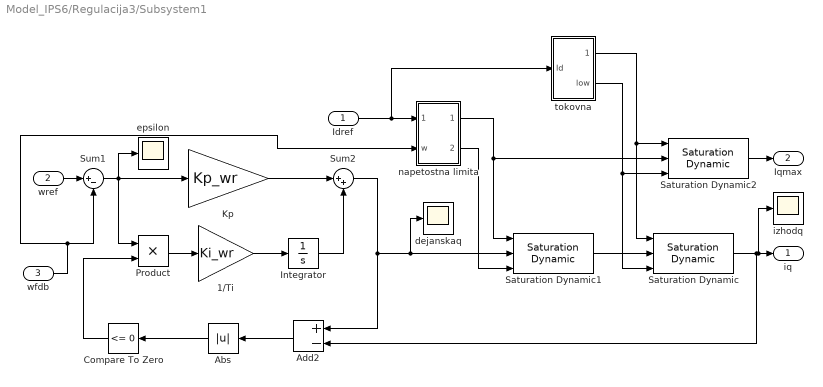
== system Model_IPS6/Regulacija3/Subsystem1 ==
  Idref : Inport
  wref : Inport  Port=2
  wfdb : Inport  Port=3
  1/Ti : Gain  Gain=Ki_wr  SaturateOnIntegerOverflow=on  OutDataTypeStr=Inherit: Same as input  ParamDataTypeStr=Inherit: Same as input
  Abs : Abs
  Add2 : Sum  Inputs=+-
  Compare To Zero : simulink/Logic and Bit Operations/Compare To Zero  relop=<=  OutDataTypeStr=boolean
  Integrator : Integrator
  Kp : Gain  Gain=Kp_wr  SaturateOnIntegerOverflow=on  OutDataTypeStr=Inherit: Same as input  ParamDataTypeStr=Inherit: Same as input
  Product : Product
  Saturation Dynamic : simulink/Discontinuities/Saturation Dynamic  OutMin=[]  OutMax=[]  OutDataTypeStr=Inherit: Same as second input  OutDataType=fixdt(1, 16)  OutScaling=2^-10  DoSatur=off
  Saturation Dynamic1 : simulink/Discontinuities/Saturation Dynamic  OutMin=[]  OutMax=[]  OutDataTypeStr=Inherit: Same as second input  OutDataType=fixdt(1, 16)  OutScaling=2^-10  DoSatur=off
  Saturation Dynamic2 : simulink/Discontinuities/Saturation Dynamic  OutMin=[]  OutMax=[]  OutDataTypeStr=Inherit: Same as second input  OutDataType=fixdt(1, 16)  OutScaling=2^-10  DoSatur=off
  Sum1 : Sum  Inputs=|+-
  Sum2 : Sum  Inputs=|++
  dejanskaq : Scope
  epsilon : Scope
  izhodq : Scope
  napetostna limita : Subsystem
  tokovna : Subsystem
  iq : Outport
  Iqmax : Outport  Port=2
  wires:
  Saturation Dynamic2/1 -> Iqmax/1
  tokovna/2(low) -> Saturation Dynamic/3, Saturation Dynamic2/3
  Sum2/1 -> Add2/1, Saturation Dynamic1/2, dejanskaq/1
  napetostna limita/1(high) -> Saturation Dynamic2/2, Saturation Dynamic1/1
  napetostna limita/2(low) -> Saturation Dynamic1/3
  Saturation Dynamic1/1 -> Saturation Dynamic/2
  tokovna/1(high) -> Saturation Dynamic/1, Saturation Dynamic2/1
  wfdb/1 -> Sum1/2, napetostna limita/2(w)
  Idref/1 -> napetostna limita/1(Idref), tokovna/1(Id)
  wref/1 -> Sum1/1
  Product/1 -> 1/Ti/1
  Compare To Zero/1 -> Product/2
  Kp/1 -> Sum2/1
  Abs/1 -> Compare To Zero/1
  Saturation Dynamic/1 -> Add2/2, iq/1, izhodq/1
  Add2/1 -> Abs/1
  Integrator/1 -> Sum2/2
  Sum1/1 -> Kp/1, Product/1, epsilon/1
  1/Ti/1 -> Integrator/1

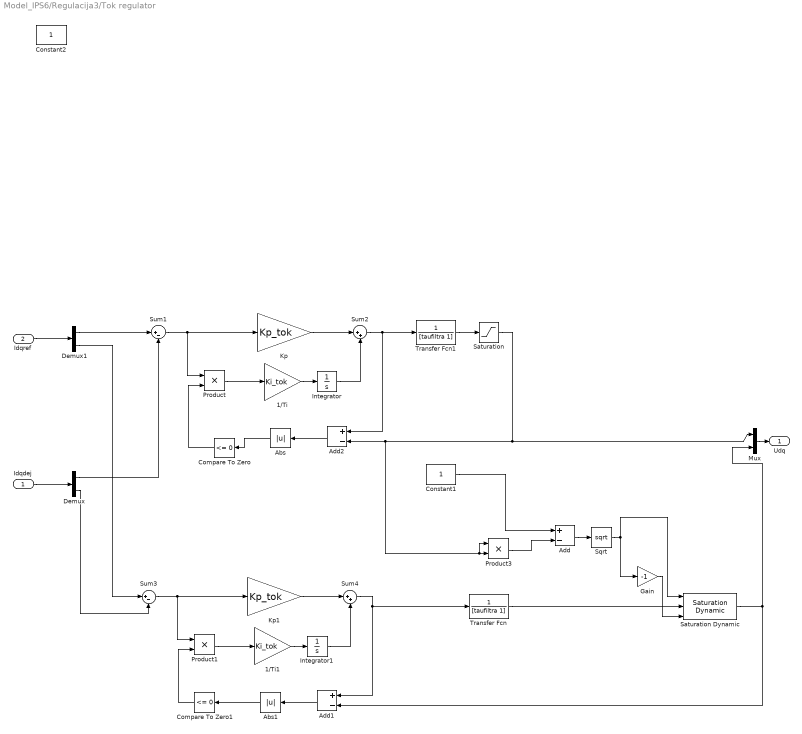
== system Model_IPS6/Regulacija3/Tok regulator ==
  Idqdej : Inport
  Idqref : Inport  Port=2
  1/Ti : Gain  Gain=Ki_tok  SaturateOnIntegerOverflow=on  OutDataTypeStr=Inherit: Same as input  ParamDataTypeStr=Inherit: Same as input
  1/Ti1 : Gain  Gain=Ki_tok  SaturateOnIntegerOverflow=on  OutDataTypeStr=Inherit: Same as input  ParamDataTypeStr=Inherit: Same as input
  Abs : Abs  ZeroCross=off
  Abs1 : Abs
  Add : Sum  Inputs=+-
  Add1 : Sum  Inputs=+-
  Add2 : Sum  Inputs=+-
  Compare To Zero : simulink/Logic and Bit Operations/Compare To Zero  relop=<=  OutDataTypeStr=boolean  ZeroCross=off
  Compare To Zero1 : simulink/Logic and Bit Operations/Compare To Zero  relop=<=  OutDataTypeStr=boolean
  Constant1 : Constant
  Constant2 : Constant
  Demux : Demux  Outputs=2
  Demux1 : Demux  Outputs=2
  Gain : Gain  Gain=-1
  Integrator : Integrator
  Integrator1 : Integrator
  Kp : Gain  Gain=Kp_tok  SaturateOnIntegerOverflow=on  OutDataTypeStr=Inherit: Same as input  ParamDataTypeStr=Inherit: Same as input
  Kp1 : Gain  Gain=Kp_tok  SaturateOnIntegerOverflow=on  OutDataTypeStr=Inherit: Same as input  ParamDataTypeStr=Inherit: Same as input
  Mux : Mux  Inputs=2
  Product : Product
  Product1 : Product
  Product3 : Product
  Saturation : Saturate  UpperLimit=0.990  LowerLimit=-0.990  ZeroCross=off
  Saturation Dynamic : simulink/Discontinuities/Saturation Dynamic  OutMin=[]  OutMax=[]  OutDataTypeStr=Inherit: Same as second input  OutDataType=fixdt(1, 16)  OutScaling=2^-10  DoSatur=off
  Sqrt : Sqrt  SaturateOnIntegerOverflow=on
  Sum1 : Sum  Inputs=|+-
  Sum2 : Sum  Inputs=|++
  Sum3 : Sum  Inputs=|+-
  Sum4 : Sum  Inputs=|++
  Transfer Fcn : TransferFcn  Denominator=[taufiltra 1]
  Transfer Fcn1 : TransferFcn  Denominator=[taufiltra 1]
  Udq : Outport
  wires:
  Transfer Fcn1/1 -> Saturation/1
  Sum2/1 -> Transfer Fcn1/1, Add2/1
  Transfer Fcn/1 -> Saturation Dynamic/2
  Sum4/1 -> Add1/1, Transfer Fcn/1
  Constant1/1 -> Add/1
  Product3/1 -> Add/2
  Sqrt/1 -> Saturation Dynamic/1, Gain/1
  Add/1 -> Sqrt/1
  Gain/1 -> Saturation Dynamic/3
  Saturation/1 -> Product3/2, Product3/1, Add2/2, Mux/1
  Demux/1 -> Sum1/2
  Demux/2 -> Sum3/2
  Idqdej/1 -> Demux/1
  Product/1 -> 1/Ti/1
  Compare To Zero/1 -> Product/2
  Abs/1 -> Compare To Zero/1
  Add2/1 -> Abs/1
  1/Ti/1 -> Integrator/1
  Demux1/1 -> Sum1/1
  Kp/1 -> Sum2/1
  Integrator/1 -> Sum2/2
  Sum1/1 -> Kp/1, Product/1
  Mux/1 -> Udq/1
  Idqref/1 -> Demux1/1
  Demux1/2 -> Sum3/1
  Sum3/1 -> Product1/1, Kp1/1
  1/Ti1/1 -> Integrator1/1
  Kp1/1 -> Sum4/1
  Saturation Dynamic/1 -> Add1/2, Mux/2
  Integrator1/1 -> Sum4/2
  Product1/1 -> 1/Ti1/1
  Compare To Zero1/1 -> Product1/2
  Add1/1 -> Abs1/1
  Abs1/1 -> Compare To Zero1/1

== system Model_IPS6/Regulacija3/Transformacije ==
  kot : Inport
  I123 : Inport  Port=2
  Udq : Inport  Port=3
  Clarke : Subsystem
  Inverzni Clarke : Subsystem
  Inverzni Park : Subsystem
  Park : Subsystem
  Idq : Outport
  U123 : Outport  Port=2
  wires:
  I123/1 -> Clarke/1(I_123)
  Udq/1 -> Inverzni Park/2(U_dq)
  Inverzni Park/1(U_ab) -> Inverzni Clarke/1(U_ab)
  Clarke/1(I_ab) -> Park/1(I_ab)
  kot/1 -> Inverzni Park/1(kot), Park/2(kot)
  Park/1(I_dq) -> Idq/1
  Inverzni Clarke/1(U_123) -> U123/1

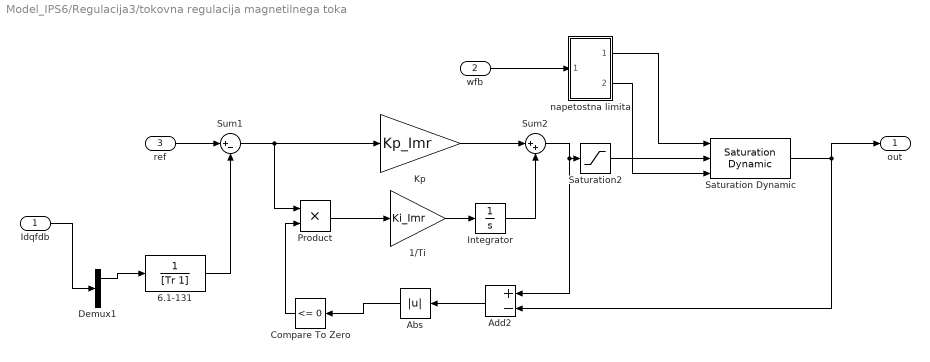
== system Model_IPS6/Regulacija3/tokovna regulacija magnetilnega toka ==
  Idqfdb : Inport
  wfb : Inport  Port=2
  ref : Inport  Port=3
  1/Ti : Gain  Gain=Ki_Imr  SaturateOnIntegerOverflow=on  OutDataTypeStr=Inherit: Same as input  ParamDataTypeStr=Inherit: Same as input
  6.1-131 : TransferFcn  Denominator=[Tr 1]
  Abs : Abs
  Add2 : Sum  Inputs=+-
  Compare To Zero : simulink/Logic and Bit Operations/Compare To Zero  relop=<=  OutDataTypeStr=boolean
  Demux1 : Demux  Outputs=2
  Integrator : Integrator
  Kp : Gain  Gain=Kp_Imr  SaturateOnIntegerOverflow=on  OutDataTypeStr=Inherit: Same as input  ParamDataTypeStr=Inherit: Same as input
  Product : Product
  Saturation Dynamic : simulink/Discontinuities/Saturation Dynamic  OutMin=[]  OutMax=[]  OutDataTypeStr=Inherit: Same as second input  OutDataType=fixdt(1, 16)  OutScaling=2^-10  DoSatur=off
  Saturation2 : Saturate  UpperLimit=Ismax  LowerLimit=0
  Sum1 : Sum  Inputs=|+-
  Sum2 : Sum  Inputs=|++
  napetostna limita : Subsystem
  out : Outport
  wires:
  Saturation Dynamic/1 -> Add2/2, out/1
  napetostna limita/2(Out2) -> Saturation Dynamic/3
  napetostna limita/1(Out1) -> Saturation Dynamic/1
  wfb/1 -> napetostna limita/1(wfb)
  Saturation2/1 -> Saturation Dynamic/2
  Idqfdb/1 -> Demux1/1
  6.1-131/1 -> Sum1/2
  Demux1/1 -> 6.1-131/1
  Kp/1 -> Sum2/1
  1/Ti/1 -> Integrator/1
  Sum1/1 -> Product/1, Kp/1
  ref/1 -> Sum1/1
  Integrator/1 -> Sum2/2
  Sum2/1 -> Saturation2/1, Add2/1
  Add2/1 -> Abs/1
  Abs/1 -> Compare To Zero/1
  Compare To Zero/1 -> Product/2
  Product/1 -> 1/Ti/1

== system Model_IPS6/TechniqueB1/Const c ==
  Id : Inport
  6.1-131 : TransferFcn  Denominator=[Tr 1]
  Scope : Scope
  Subtract : Sum  Inputs=+-
  Transfer Fcn : TransferFcn  Denominator=[0.2 1]
  konstanta c : Gain  Gain=Lm^2/Lr
  c : Outport
  Imr : Outport  Port=2
  wires:
  Id/1 -> Subtract/2, 6.1-131/1
  6.1-131/1 -> Imr/1, Subtract/1
  Subtract/1 -> konstanta c/1
  konstanta c/1 -> Transfer Fcn/1
  Transfer Fcn/1 -> Scope/1, c/1

== system Model_IPS6/Asinhronski stroj1/Clarke/ABC_ab1 ==
  A : Inport
  B : Inport  Port=2
  C : Inport  Port=3
  Gain1 : Gain  Gain=2
  Gain2 : Gain
  Gain24 : Gain  Gain=sqrt(3)/3
  Sum11 : Sum
  Terminator : Terminator
  alfa : Outport
  beta : Outport  Port=2
  wires:
  C/1 -> Terminator/1
  Gain1/1 -> Sum11/2
  B/1 -> Gain1/1
  Gain24/1 -> beta/1
  Gain2/1 -> alfa/1
  Sum11/1 -> Gain24/1
  A/1 -> Sum11/1, Gain2/1

== system Model_IPS6/Asinhronski stroj1/Inverzni Clarke/ab_ABC ==
  alfa : Inport
  beta : Inport  Port=2
  Gain1 : Gain
  Gain2 : Gain  Gain=-0.5
  Gain25 : Gain  Gain=sqrt(3)/2
  Gain3 : Gain  Gain=sqrt(3)/2
  Gain4 : Gain  Gain=0.5
  Sum10 : Sum
  Sum11 : Sum  Inputs=--
  A : Outport
  B : Outport  Port=2
  C : Outport  Port=3
  wires:
  Gain3/1 -> Sum11/2
  beta/1 -> Gain25/1, Gain3/1
  Gain4/1 -> Sum11/1
  Gain25/1 -> Sum10/2
  Gain2/1 -> Sum10/1
  alfa/1 -> Gain1/1, Gain2/1, Gain4/1
  Gain1/1 -> A/1
  Sum10/1 -> B/1
  Sum11/1 -> C/1

== system Model_IPS6/Asinhronski stroj1/Mehanika/eq 2.19 ==
  M : Inport
  Gain1 : Gain  Gain=1/J
  Integrator : Integrator
  wr : Outport
  wires:
  Integrator/1 -> wr/1
  M/1 -> Gain1/1
  Gain1/1 -> Integrator/1

== system Model_IPS6/Asinhronski stroj1/napetostni dq model/eq 5.35 ==
  Imr : Inport
  Isq : Inport  Port=2
  Gain : Gain  Gain=3*pp/2
  Gain2 : Gain  Gain=Lm*Lm/Lr
  Product : Product  RndMeth=Zero
  Mel : Outport
  wires:
  Gain/1 -> Gain2/1
  Gain2/1 -> Mel/1
  Product/1 -> Gain/1
  Isq/1 -> Product/2
  Imr/1 -> Product/1

== system Model_IPS6/Asinhronski stroj1/napetostni dq model/eq 5.39 ==
  Isd : Inport
  Gain : Gain  Gain=1/Tr
  Integrator : Integrator  InitialCondition=1e-3
  Sum : Sum  Inputs=|+-
  Imr : Outport
  dImr/dt : Outport  Port=2
  wires:
  Gain/1 -> dImr/dt/1, Integrator/1
  Sum/1 -> Gain/1
  Integrator/1 -> Sum/2, Imr/1
  Isd/1 -> Sum/1

== system Model_IPS6/Asinhronski stroj1/napetostni dq model/eq 5.40 ==
  Imr : Inport
  Isq : Inport  Port=2
  wr_el : Inport  Port=3
  Divide : Product  Inputs=*/
  Gain2 : Gain  Gain=Tr
  Saturation : Saturate  UpperLimit=2*pi*50  LowerLimit=-2*pi*50
  Sum : Sum  Inputs=|++
  wmr : Outport
  wires:
  Saturation/1 -> Sum/1
  Sum/1 -> wmr/1
  wr_el/1 -> Sum/2
  Divide/1 -> Saturation/1  "ws"
  Gain2/1 -> Divide/2
  Imr/1 -> Gain2/1
  Isq/1 -> Divide/1

== system Model_IPS6/Asinhronski stroj1/napetostni dq model/eq 5.46 ==
  Usd : Inport
  dImr/dt : Inport  Port=2
  Isq : Inport  Port=3
  wmr : Inport  Port=4
  Gain : Gain  Gain=1/(sigma*Ls)
  Gain1 : Gain  Gain=Rs
  Gain2 : Gain  Gain=(1-sigma)*Ls
  Gain3 : Gain  Gain=sigma*Ls
  Integrator : Integrator
  Product : Product  RndMeth=Zero
  Sum : Sum  Inputs=+--+
  Isd : Outport
  wires:
  Gain3/1 -> Sum/4
  Product/1 -> Gain3/1
  Isq/1 -> Product/1
  wmr/1 -> Product/2
  Gain2/1 -> Sum/3
  dImr/dt/1 -> Gain2/1
  Gain1/1 -> Sum/2
  Usd/1 -> Sum/1
  Sum/1 -> Gain/1
  Gain/1 -> Integrator/1
  Integrator/1 -> Gain1/1, Isd/1

== system Model_IPS6/Asinhronski stroj1/napetostni dq model/eq 5.47 ==
  Usq : Inport
  Imr : Inport  Port=2
  Isd : Inport  Port=3
  wmr : Inport  Port=4
  Gain : Gain  Gain=1/(sigma*Ls)
  Gain1 : Gain  Gain=Rs
  Gain2 : Gain  Gain=(1-sigma)*Ls
  Gain3 : Gain  Gain=sigma*Ls
  Integrator : Integrator
  Product : Product  RndMeth=Zero
  Product1 : Product  RndMeth=Zero
  Sum : Sum  Inputs=+---
  Isq : Outport
  wires:
  Gain3/1 -> Sum/4
  Product1/1 -> Gain3/1
  Isd/1 -> Product1/2
  Gain2/1 -> Sum/3
  Product/1 -> Gain2/1
  wmr/1 -> Product1/1, Product/2
  Imr/1 -> Product/1
  Gain1/1 -> Sum/2
  Usq/1 -> Sum/1
  Sum/1 -> Gain/1
  Gain/1 -> Integrator/1
  Integrator/1 -> Gain1/1, Isq/1

== system Model_IPS6/Asinhronski stroj2/Clarke/ABC_ab1 ==
  A : Inport
  B : Inport  Port=2
  C : Inport  Port=3
  Gain1 : Gain  Gain=2
  Gain2 : Gain
  Gain24 : Gain  Gain=sqrt(3)/3
  Sum11 : Sum
  Terminator : Terminator
  alfa : Outport
  beta : Outport  Port=2
  wires:
  A/1 -> Gain2/1, Sum11/1
  Sum11/1 -> Gain24/1
  Gain2/1 -> alfa/1
  Gain24/1 -> beta/1
  B/1 -> Gain1/1
  Gain1/1 -> Sum11/2
  C/1 -> Terminator/1

== system Model_IPS6/Asinhronski stroj2/Inverzni Clarke/ab_ABC ==
  alfa : Inport
  beta : Inport  Port=2
  Gain1 : Gain
  Gain2 : Gain  Gain=-0.5
  Gain25 : Gain  Gain=sqrt(3)/2
  Gain3 : Gain  Gain=sqrt(3)/2
  Gain4 : Gain  Gain=0.5
  Sum10 : Sum
  Sum11 : Sum  Inputs=--
  A : Outport
  B : Outport  Port=2
  C : Outport  Port=3
  wires:
  Sum11/1 -> C/1
  Sum10/1 -> B/1
  Gain1/1 -> A/1
  alfa/1 -> Gain4/1, Gain2/1, Gain1/1
  Gain2/1 -> Sum10/1
  Gain25/1 -> Sum10/2
  Gain4/1 -> Sum11/1
  beta/1 -> Gain3/1, Gain25/1
  Gain3/1 -> Sum11/2

== system Model_IPS6/Asinhronski stroj2/Mehanika/eq 2.19 ==
  M : Inport
  Gain1 : Gain  Gain=1/J
  Integrator : Integrator
  wr : Outport
  wires:
  Gain1/1 -> Integrator/1
  M/1 -> Gain1/1
  Integrator/1 -> wr/1

== system Model_IPS6/Asinhronski stroj2/napetostni dq model/eq 5.35 ==
  Imr : Inport
  Isq : Inport  Port=2
  Gain : Gain  Gain=3*pp/2
  Gain2 : Gain  Gain=Lm*Lm/Lr
  Product : Product  RndMeth=Zero
  Mel : Outport
  wires:
  Imr/1 -> Product/1
  Isq/1 -> Product/2
  Product/1 -> Gain/1
  Gain2/1 -> Mel/1
  Gain/1 -> Gain2/1

== system Model_IPS6/Asinhronski stroj2/napetostni dq model/eq 5.39 ==
  Isd : Inport
  Gain : Gain  Gain=1/Tr
  Integrator : Integrator  InitialCondition=1e-3
  Sum : Sum  Inputs=|+-
  Imr : Outport
  dImr/dt : Outport  Port=2
  wires:
  Isd/1 -> Sum/1
  Integrator/1 -> Imr/1, Sum/2
  Sum/1 -> Gain/1
  Gain/1 -> Integrator/1, dImr/dt/1

== system Model_IPS6/Asinhronski stroj2/napetostni dq model/eq 5.40 ==
  Imr : Inport
  Isq : Inport  Port=2
  wr_el : Inport  Port=3
  Divide : Product  Inputs=*/
  Gain2 : Gain  Gain=Tr
  Saturation : Saturate  UpperLimit=2*pi*50  LowerLimit=-2*pi*50
  Sum : Sum  Inputs=|++
  wmr : Outport
  wires:
  Isq/1 -> Divide/1
  Imr/1 -> Gain2/1
  Gain2/1 -> Divide/2
  Divide/1 -> Saturation/1  "ws"
  wr_el/1 -> Sum/2
  Sum/1 -> wmr/1
  Saturation/1 -> Sum/1

== system Model_IPS6/Asinhronski stroj2/napetostni dq model/eq 5.46 ==
  Usd : Inport
  dImr/dt : Inport  Port=2
  Isq : Inport  Port=3
  wmr : Inport  Port=4
  Gain : Gain  Gain=1/(sigma*Ls)
  Gain1 : Gain  Gain=Rs
  Gain2 : Gain  Gain=(1-sigma)*Ls
  Gain3 : Gain  Gain=sigma*Ls
  Integrator : Integrator
  Product : Product  RndMeth=Zero
  Sum : Sum  Inputs=+--+
  Isd : Outport
  wires:
  Integrator/1 -> Isd/1, Gain1/1
  Gain/1 -> Integrator/1
  Sum/1 -> Gain/1
  Usd/1 -> Sum/1
  Gain1/1 -> Sum/2
  dImr/dt/1 -> Gain2/1
  Gain2/1 -> Sum/3
  wmr/1 -> Product/2
  Isq/1 -> Product/1
  Product/1 -> Gain3/1
  Gain3/1 -> Sum/4

== system Model_IPS6/Asinhronski stroj2/napetostni dq model/eq 5.47 ==
  Usq : Inport
  Imr : Inport  Port=2
  Isd : Inport  Port=3
  wmr : Inport  Port=4
  Gain : Gain  Gain=1/(sigma*Ls)
  Gain1 : Gain  Gain=Rs
  Gain2 : Gain  Gain=(1-sigma)*Ls
  Gain3 : Gain  Gain=sigma*Ls
  Integrator : Integrator
  Product : Product  RndMeth=Zero
  Product1 : Product  RndMeth=Zero
  Sum : Sum  Inputs=+---
  Isq : Outport
  wires:
  Integrator/1 -> Isq/1, Gain1/1
  Gain/1 -> Integrator/1
  Sum/1 -> Gain/1
  Usq/1 -> Sum/1
  Gain1/1 -> Sum/2
  Imr/1 -> Product/1
  wmr/1 -> Product/2, Product1/1
  Product/1 -> Gain2/1
  Gain2/1 -> Sum/3
  Isd/1 -> Product1/2
  Product1/1 -> Gain3/1
  Gain3/1 -> Sum/4

== system Model_IPS6/Regulacija1/Regulacija navora/Limita q toka ==
  Idref : Inport
  w : Inport  Port=2
  Iq : Inport  Port=3
  0 : Constant  Value=0
  Saturation napetost : simulink/Discontinuities/Saturation Dynamic  OutMin=[]  OutMax=[]  OutDataTypeStr=Inherit: Same as second input  OutDataType=fixdt(1, 16)  OutScaling=2^-10  DoSatur=off
  Saturation presek : simulink/Discontinuities/Saturation Dynamic  OutMin=[]  OutMax=[]  OutDataTypeStr=Inherit: Same as second input  OutDataType=fixdt(1, 16)  OutScaling=2^-10  DoSatur=off
  Saturation tok : simulink/Discontinuities/Saturation Dynamic  OutMin=[]  OutMax=[]  OutDataTypeStr=Inherit: Same as second input  OutDataType=fixdt(1, 16)  OutScaling=2^-10  DoSatur=off
  Scope : Scope  NumInputPorts=3
  Scope1 : Scope
  napetostna limita : Subsystem
  tokovna : Subsystem
  Out1 : Outport
  Iq_lim : Outport  Port=2
  wires:
  w/1 -> napetostna limita/2(w)
  napetostna limita/1(high) -> Saturation presek/1, Saturation napetost/1
  Idref/1 -> tokovna/1(Id), napetostna limita/1(Idref)
  tokovna/2(low) -> Saturation tok/3
  tokovna/1(high) -> Saturation presek/2, Saturation tok/1
  Saturation presek/1 -> Scope1/1, Out1/1
  napetostna limita/2(low) -> Saturation napetost/3
  Saturation tok/1 -> Scope/2, Saturation napetost/2
  Iq/1 -> Scope/1, Saturation tok/2
  Saturation napetost/1 -> Scope/3, Iq_lim/1
  0/1 -> Saturation presek/3

== system Model_IPS6/Regulacija1/Tok regulator/Subsystem ==
  Ud : Inport
  Uq : Inport  Port=2
  Add : Sum  Inputs=+-
  Constant1 : Constant
  Gain : Gain  Gain=-1
  Product3 : Product
  Saturation Dynamic : simulink/Discontinuities/Saturation Dynamic  OutMin=[]  OutMax=[]  OutDataTypeStr=Inherit: Same as second input  OutDataType=fixdt(1, 16)  OutScaling=2^-10  DoSatur=off
  Scope : Scope  NumInputPorts=2
  Sqrt : Sqrt  SaturateOnIntegerOverflow=on
  Uq_lim : Outport
  wires:
  Ud/1 -> Product3/1, Product3/2
  Uq/1 -> Scope/1, Saturation Dynamic/2
  Saturation Dynamic/1 -> Scope/2, Uq_lim/1
  Constant1/1 -> Add/1
  Gain/1 -> Saturation Dynamic/3
  Product3/1 -> Add/2
  Add/1 -> Sqrt/1
  Sqrt/1 -> Gain/1, Saturation Dynamic/1

== system Model_IPS6/Regulacija1/Transformacije/Clarke ==
  I_123 : Inport
  ABC_ab1 : Subsystem
  Demux : Demux  Outputs=3
  Mux : Mux  Inputs=2
  I_ab : Outport
  wires:
  Mux/1 -> I_ab/1
  ABC_ab1/2(beta) -> Mux/2
  ABC_ab1/1(alfa) -> Mux/1
  Demux/3 -> ABC_ab1/3(C)
  Demux/2 -> ABC_ab1/2(B)
  Demux/1 -> ABC_ab1/1(A)
  I_123/1 -> Demux/1

== system Model_IPS6/Regulacija1/Transformacije/Inverzni Clarke ==
  U_ab : Inport
  Demux : Demux  Outputs=2
  Mux : Mux  Inputs=3
  ab_ABC : Subsystem
  U_123 : Outport
  wires:
  ab_ABC/3(C) -> Mux/3
  ab_ABC/2(B) -> Mux/2
  ab_ABC/1(A) -> Mux/1
  Demux/2 -> ab_ABC/2(beta)
  Demux/1 -> ab_ABC/1(alfa)
  U_ab/1 -> Demux/1
  Mux/1 -> U_123/1

== system Model_IPS6/Regulacija1/Transformacije/Inverzni Park ==
  kot : Inport
  U_dq : Inport  Port=2
  Demux : Demux  Outputs=2
  Mux : Mux  Inputs=2
  "Sum1 " : Sum  Inputs=+-  SaturateOnIntegerOverflow=on  InputSameDT=on  OutDataTypeStr=Inherit: Same as first input
  Sum2 : Sum  SaturateOnIntegerOverflow=on  InputSameDT=on  OutDataTypeStr=Inherit: Same as first input
  cos : Fcn  Expr=cos(u)
  sin : Fcn  Expr=sin(u)
  x_d*cos : Product  SaturateOnIntegerOverflow=on  RndMeth=Zero  InputSameDT=on  OutDataTypeStr=Inherit: Same as first input
  x_d*sin : Product  SaturateOnIntegerOverflow=on  RndMeth=Zero  InputSameDT=on  OutDataTypeStr=Inherit: Same as first input
  x_q*cos : Product  SaturateOnIntegerOverflow=on  RndMeth=Zero  InputSameDT=on  OutDataTypeStr=Inherit: Same as first input
  "x_q*sin " : Product  SaturateOnIntegerOverflow=on  RndMeth=Zero  InputSameDT=on  OutDataTypeStr=Inherit: Same as first input
  U_ab : Outport
  wires:
  Mux/1 -> U_ab/1
  U_dq/1 -> Demux/1
  Demux/1 -> x_d*sin/1, x_d*cos/1
  Demux/2 -> "x_q*sin "/1, x_q*cos/1
  cos/1 -> x_q*cos/2, x_d*cos/2
  sin/1 -> "x_q*sin "/2, x_d*sin/2
  x_d*cos/1 -> "Sum1 "/1
  "x_q*sin "/1 -> "Sum1 "/2
  x_q*cos/1 -> Sum2/2
  x_d*sin/1 -> Sum2/1
  "Sum1 "/1 -> Mux/1
  Sum2/1 -> Mux/2
  kot/1 -> cos/1, sin/1

== system Model_IPS6/Regulacija1/Transformacije/Park ==
  I_ab : Inport
  kot : Inport  Port=2
  Demux : Demux  Outputs=2
  Mux : Mux  Inputs=2
  "Sum1 " : Sum  SaturateOnIntegerOverflow=on  InputSameDT=on  OutDataTypeStr=Inherit: Same as first input
  Sum2 : Sum  Inputs=-+  SaturateOnIntegerOverflow=on  InputSameDT=on  OutDataTypeStr=Inherit: Same as first input
  cos : Fcn  Expr=cos(u)
  sin : Fcn  Expr=sin(u)
  x_a*cos : Product  SaturateOnIntegerOverflow=on  RndMeth=Zero  InputSameDT=on  OutDataTypeStr=Inherit: Same as first input
  x_a*sin : Product  SaturateOnIntegerOverflow=on  RndMeth=Zero  InputSameDT=on  OutDataTypeStr=Inherit: Same as first input
  x_b*cos : Product  SaturateOnIntegerOverflow=on  RndMeth=Zero  InputSameDT=on  OutDataTypeStr=Inherit: Same as first input
  "x_b*sin " : Product  SaturateOnIntegerOverflow=on  RndMeth=Zero  InputSameDT=on  OutDataTypeStr=Inherit: Same as first input
  I_dq : Outport
  wires:
  Mux/1 -> I_dq/1
  I_ab/1 -> Demux/1
  Demux/1 -> x_a*sin/1, x_a*cos/1
  Demux/2 -> "x_b*sin "/1, x_b*cos/1
  cos/1 -> x_b*cos/2, x_a*cos/2
  sin/1 -> "x_b*sin "/2, x_a*sin/2
  x_a*cos/1 -> "Sum1 "/1
  "x_b*sin "/1 -> "Sum1 "/2
  x_b*cos/1 -> Sum2/2
  x_a*sin/1 -> Sum2/1
  "Sum1 "/1 -> Mux/1
  Sum2/1 -> Mux/2
  kot/1 -> cos/1, sin/1

== system Model_IPS6/Regulacija1/tokovna regulacija magnetilnega toka/napetostna limita ==
  wfb : Inport
  Abs : Abs
  Add1 : Sum
  Constant : Constant  Value=0.0000001
  Constant1 : Constant  Value=Udc/Ls
  Divide : Product  Inputs=*/
  Gain : Gain  Gain=-1
  Out1 : Outport
  Out2 : Outport  Port=2
  wires:
  Add1/1 -> Divide/2
  Divide/1 -> Out1/1, Gain/1
  Constant1/1 -> Divide/1
  Constant/1 -> Add1/2
  Gain/1 -> Out2/1
  wfb/1 -> Abs/1
  Abs/1 -> Add1/1

== system Model_IPS6/Regulacija3/Subsystem1/napetostna limita ==
  Idref : Inport
  w : Inport  Port=2
  Abs : Abs
  Add1 : Sum  Inputs=-+
  Constant : Constant
  Divide : Product  Inputs=*/
  Gain : Gain  Gain=-1
  Product2 : Product
  Product3 : Product
  Sqrt : Sqrt  SaturateOnIntegerOverflow=on
  To Workspace1 : ToWorkspace  VariableName=b2  SampleTime=-1
      settings: Decimation=3  Save2DSignal=2-D array (concatenate along first dimension)
  To Workspace7 : ToWorkspace  VariableName=a2  SampleTime=-1
      settings: Decimation=3  Save2DSignal=2-D array (concatenate along first dimension)
  a : Subsystem
  b : Subsystem
  high : Outport
  low : Outport  Port=2
  wires:
  Abs/1 -> high/1, Gain/1
  a/1(Out1) -> Divide/2, To Workspace7/1
  Gain/1 -> low/1
  b/1(Out1) -> Product3/2, To Workspace1/1
  Add1/1 -> Sqrt/1
  Product2/1 -> Add1/1
  Product3/1 -> Abs/1
  w/1 -> a/1(In1), b/1(In1)
  Constant/1 -> Add1/2
  Divide/1 -> Product2/2, Product2/1
  Idref/1 -> Divide/1
  Sqrt/1 -> Product3/1

== system Model_IPS6/Regulacija3/Subsystem1/tokovna ==
  Id : Inport
  Abs : Abs
  Constant : Constant  Value=Ismax^2
  Gain2 : Gain  Gain=-1
  Product1 : Product
  Sqrt : Sqrt  SaturateOnIntegerOverflow=on
  Subtract : Sum  Inputs=+-
  high : Outport
  low : Outport  Port=2
  wires:
  Abs/1 -> high/1, Gain2/1
  Subtract/1 -> Sqrt/1
  Product1/1 -> Subtract/2
  Constant/1 -> Subtract/1
  Gain2/1 -> low/1
  Id/1 -> Product1/1, Product1/2
  Sqrt/1 -> Abs/1

== system Model_IPS6/Regulacija3/Transformacije/Clarke ==
  I_123 : Inport
  ABC_ab1 : Subsystem
  Demux : Demux  Outputs=3
  Mux : Mux  Inputs=2
  I_ab : Outport
  wires:
  I_123/1 -> Demux/1
  Demux/1 -> ABC_ab1/1(A)
  Demux/2 -> ABC_ab1/2(B)
  Demux/3 -> ABC_ab1/3(C)
  ABC_ab1/1(alfa) -> Mux/1
  ABC_ab1/2(beta) -> Mux/2
  Mux/1 -> I_ab/1
